simulink model "example_simulation"  (R2024b)
settings: Solver=FixedStepAuto  StartTime=0.0  StopTime=10.0  FixedStep=5/1000  RelTol=1e-3
settings Model: DataDictionary=example_datadict.sldd  Creator=zhanfuyu  LastModifiedBy=CETCA
settings OptimizationCC: ReuseModelBlockBuffer=off
settings RTWCC: GPUComputeCapability=3.5

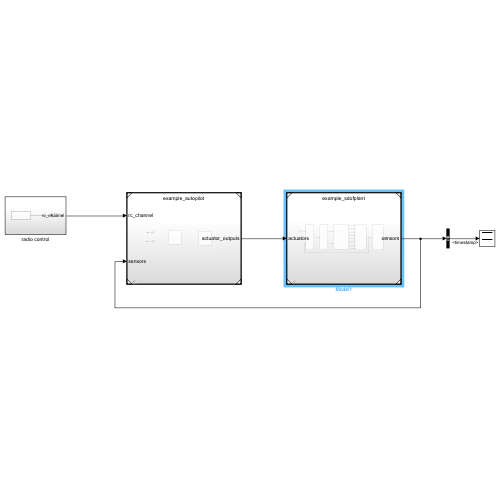
[thumbnail: Simulink's stored preview of the top-level diagram]
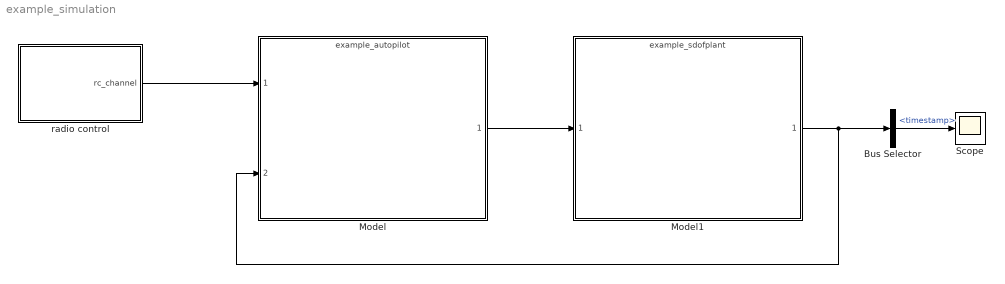
== system example_simulation ==
  Bus Selector : BusSelector  OutputSignals=gps.timestamp
  Model : ModelReference  ModelNameDialog=example_autopilot.slx  SimulationMode=Normal  ModelReferenceVersion=5.7
  Model1 : ModelReference  ModelNameDialog=example_sdofplant.slx  SimulationMode=Normal  ModelReferenceVersion=5.73
  Scope : Scope
  radio control : Subsystem
  wires:
  radio control/1(rc_channel) -> Model/1
  Bus Selector/1 -> Scope/1  "<timestamp>"
  Model1/1 -> Bus Selector/1, Model/2
  Model/1 -> Model1/1

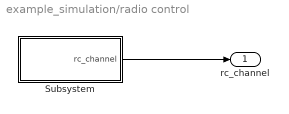
== system example_simulation/radio control ==
  Subsystem : Subsystem
  rc_channel : Outport  OutDataTypeStr=Bus: rc_channels_s
  wires:
  Subsystem/1(rc_channel) -> rc_channel/1

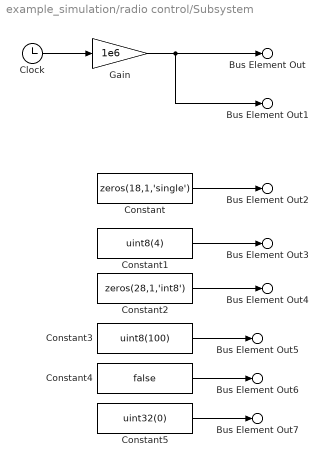
== system example_simulation/radio control/Subsystem ==
  Clock : Clock
  Constant : Constant  Value=zeros(18,1,'single')
  Constant1 : Constant  Value=uint8(4)
  Constant2 : Constant  Value=zeros(28,1,'int8')
  Constant3 : Constant  Value=uint8(100)
  Constant4 : Constant  Value=false
  Constant5 : Constant  Value=uint32(0)
  Gain : Gain  Gain=1e6  OutDataTypeStr=uint64
  Bus Element Out : Outport  PortName=rc_channel  Element=timestamp
  Bus Element Out1 : Outport  PortName=rc_channel  Element=timestamp_last_valid
  Bus Element Out2 : Outport  PortName=rc_channel  Element=channels
  Bus Element Out3 : Outport  PortName=rc_channel  Element=channel_count
  Bus Element Out4 : Outport  PortName=rc_channel  Element=function
  Bus Element Out5 : Outport  PortName=rc_channel  Element=rssi
  Bus Element Out6 : Outport  PortName=rc_channel  Element=signal_lost
  Bus Element Out7 : Outport  PortName=rc_channel  Element=frame_drop_count
  wires:
  Clock/1 -> Gain/1
  Gain/1 -> Bus Element Out1/1, Bus Element Out/1
  Constant/1 -> Bus Element Out2/1
  Constant1/1 -> Bus Element Out3/1
  Constant2/1 -> Bus Element Out4/1
  Constant3/1 -> Bus Element Out5/1
  Constant4/1 -> Bus Element Out6/1
  Constant5/1 -> Bus Element Out7/1
